simulink model "Simulink_3"  (R2013b)
settings: Solver=ode45  StartTime=0.0  StopTime=50.0  RelTol=1e-5
libraries: simulink x1
settings Model: Creator=99900361  LastModifiedBy=99900361
settings DataIOCC: SignalLoggingSaveFormat=ModelDataLogs  SignalLoggingName=sigsOut
settings DebuggingCC: SaveWithParameterizedLinksMsg=none  SignalResolutionControl=TryResolveAllWithWarning  SolverPrmCheckMsg=none  MultiTaskDSMMsg=warning  MultiTaskCondExecSysMsg=none  StrictBusMsg=None
settings HardwareCC: TargetUnknown=on
settings RTWCC: IncludeERTFirstTime=on
settings GRTTargetCC: CombineOutputUpdateFcns=off  GRTInterface=on

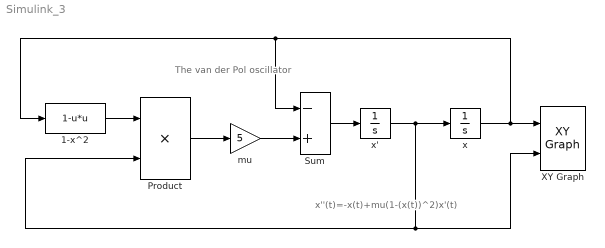
== system Simulink_3 ==
  note: x''(t)=-x(t)+mu(1-(x(t))^2)x'(t)
  note: The van der Pol oscillator
  1-x^2 : Fcn  Expr=1-u*u
  Product : Product  SaturateOnIntegerOverflow=on  OutDataTypeStr=Inherit: Same as first input
  Sum : Sum  Inputs=-+  SaturateOnIntegerOverflow=on
  XY Graph : simulink/Sinks/XY Graph  xmin=-3  xmax=3  ymin=-10  ymax=10  st=-1
  mu : Gain  Gain=5  SaturateOnIntegerOverflow=on  OutDataTypeStr=Inherit: Same as input  ParamDataTypeStr=Inherit: Same as input
  x : Integrator  InitialCondition=2
  x' : Integrator
  wires:
  mu/1 -> Sum/2
  Sum/1 -> x'/1
  x'/1 -> x/1, Product/2, XY Graph/2
  x/1 -> Sum/1, 1-x^2/1, XY Graph/1
  Product/1 -> mu/1
  1-x^2/1 -> Product/1
